simulink model "SerExample"  (R2019b)
settings: Solver=FixedStepAuto  StartTime=0.0  StopTime=inf  FixedStep=1e-3  RelTol=1e-3  EnableMultiTasking=on
libraries: frdmk64flib x6, nucleoutilitieslib x1
settings Model: ExtModeTrigDuration=5  Creator=shahv10  LastModifiedBy=shahv10
settings OptimizationCC: EnhancedBackFolding=on  PassReuseOutputArgsAs=Individual arguments  ZeroExternalMemoryAtStartup=off  ZeroInternalMemoryAtStartup=off  MaxStackSize=64  OptimizeBlockOrder=speed  DifferentSizesBufferReuse=on  OptimizationCustomize=off  EfficientTunableParamExpr=on
settings DebuggingCC: ParameterTunabilityLossMsg=error
settings HardwareCC: ProdBitPerPointer=32  ProdBitPerSizeT=32  ProdBitPerPtrDiffT=32  ProdLargestAtomicInteger=Long  ProdLargestAtomicFloat=Double  ProdWordSize=32  ProdHWDeviceType=ARM Compatible->ARM Cortex  UseEmbeddedCoderFeatures=off
settings SFSimCC: MATLABDynamicMemAlloc=off
settings RTWCC: SystemTargetFile=ert.tlc  HardwareBoard=NXP FRDM-K64F  TLCOptions="-aInlineSetEventsForThisBaseRateFcn=TLC_FALSE -aSuppressMultiTaskScheduler=TLC_FALSE  -aRateBasedStepFcn=0"  TemplateMakefile=ert_default_tmf  GenerateReport=on  Toolchain=GNU Tools for ARM Embedded Processors  IncludeHyperlinkInReport=on  LaunchReport=on  GenerateTraceInfo=on  GenerateTraceReport=on  GenerateTraceReportSl=on  GenerateTraceReportSf=on  GenerateTraceReportEml=on
settings CodeAppCC: ForceParamTrailComments=on  IgnoreCustomStorageClasses=off  OperatorAnnotations=on  SimulinkDataObjDesc=on  SFDataObjDesc=on  InsertBlockDesc=on
settings ERTTargetCC: SupportNonInlinedSFcns=on

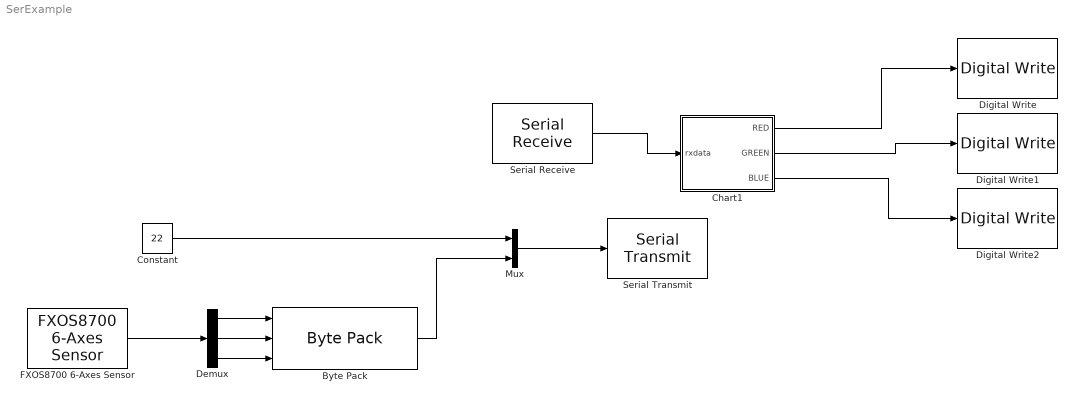
== system SerExample ==
  Byte Pack : nucleoutilitieslib/Byte Pack  datatypes={'double','double','double'}  byteAlign=1  blockPlatform=nucleo
      settings: SourceProductName=Embedded Coder Support Package for ARM Cortex-A Processors  SourceProductBaseCode=ECCORTEXA
  Chart1 : Stateflow chart  BlockKeywords=__PRM__SERIALIZED__DATA__:Stateflow Chart,Stateflow Diagram  TreatAsAtomicUnit=on
  Constant : Constant  Value=22  OutDataTypeStr=uint8
  Demux : Demux  Outputs=3
  Digital Write : frdmk64flib/Digital Write  Whichpin=RED_LED
      settings: SourceProductName=Simulink Coder Support Package for NXP FRDM-K64F Board
  Digital Write1 : frdmk64flib/Digital Write  Whichpin=GREEN_LED
      settings: SourceProductName=Simulink Coder Support Package for NXP FRDM-K64F Board
  Digital Write2 : frdmk64flib/Digital Write  Whichpin=BLUE_LED
      settings: SourceProductName=Simulink Coder Support Package for NXP FRDM-K64F Board
  FXOS8700 6-Axes Sensor : frdmk64flib/FXOS8700 6-Axes Sensor  Activesensor=Accelerometer only  ODR=400Hz  HybridODR=400Hz  Accelfullrange=-8g to +8g  SampleTime=1
      settings: SourceProductName=Simulink Coder Support Package for NXP FRDM-K64F Board
  Mux : Mux  Inputs=2
  Serial Receive : frdmk64flib/Serial Receive  SCIModule=0  Baudrate=uint32(9600)  Parity=None  StopBits=1  HardwareFlowControl=None  ByteOrder=LittleEndian  DataType=uint8  DataLength=4  BlockingMode=off  OutputStatus=off  SampleTime=-1
      settings: SourceProductName=Simulink Coder Support Package for NXP FRDM-K64F Board
  Serial Transmit : frdmk64flib/Serial Transmit  SCIModule=0  Baudrate=uint32(9600)  Parity=None  StopBits=1  HardwareFlowControl=None  ByteOrder=LittleEndian  BlockingMode=on  OutputStatus=off
      settings: SourceProductName=Simulink Coder Support Package for NXP FRDM-K64F Board
  wires:
  Serial Receive/1 -> Chart1/1(rxdata)
  Chart1/1(RED) -> Digital Write/1
  Chart1/2(GREEN) -> Digital Write1/1
  Chart1/3(BLUE) -> Digital Write2/1
  Constant/1 -> Mux/1
  Mux/1 -> Serial Transmit/1
  Byte Pack/1 -> Mux/2
  FXOS8700 6-Axes Sensor/1 -> Demux/1
  Demux/1 -> Byte Pack/1
  Demux/2 -> Byte Pack/2
  Demux/3 -> Byte Pack/3

== stateflow chart SerExample/Chart1 ==
  settings: executeAtInitialization=1
  state INIT
    entry:
    RED=1;
    GREEN=0;
    BLUE=0;
  state SET_LEDs
    entry:
    RED=rxdata(2);
    GREEN=rxdata(3);
    BLUE=rxdata(4);
  state IDLE
  SET_LEDs -> IDLE
  (default) -> INIT
  INIT -> IDLE
  IDLE -> SET_LEDs : [rxdata(1) == hex2dec("16")]
  data: RED output uint8; GREEN output uint8; BLUE output uint8; rxdata input uint8
